simulink model "AUV_2DoF"  (R2020b)
settings: Solver=VariableStepAuto  StartTime=0.0  StopTime=60  RelTol=1e-3
libraries: pid_lib x4
settings Model: Creator=shanerutherford  LastModifiedBy=shanerutherford

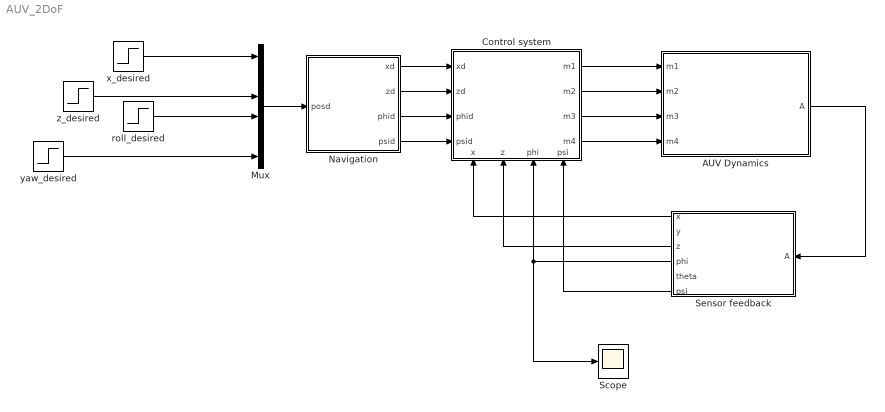
== system AUV_2DoF ==
  AUV Dynamics : Subsystem
  Control system : Subsystem
      settings: PortSchema="{\"entries\":[{\"content\":{\"sides\":[{\"content\":{\"connectorIds\":[\"In1\",\"In2\",\"In3\",\"In4\"]},\"type\":\"ConnectorPlacement.EquallySpacedRectSide\",\"uuid\":\"3eb5b42b-7b52-486e-935e-7444b7a9c48d\"},{\"content\":{\"connectorIds\":[\"Out1\",\"Out2\",\"Out3\",\"Out4\"],\"side\":\"RIGHT\"},\"type\":\"ConnectorPlacement.EquallySpacedRectSide\",\"uuid\":\"c474b75f-63e2-42a7-9927-f23487fa052b\"},{\"content\":{\"connectorIds\":[],\"side\":\"TOP\"},\"type\":\"ConnectorPlacement.EquallySpacedRectSide\",\"uuid\":\"fca6ae17-6a90-49a5-80ec-8d57e94c626d\"},{\"content\":{\"connectorIds\":[\"In5\",\"In6\",\"In7\",\"In8\"],\"side\":\"BOTTOM\"},\"type\":\"ConnectorPlacement.EquallySpacedRectSide\",\"uuid\":\"7c03cb94-1735-4782-aac2-3eb76e3c70ce\"},{\"content\":{\"connectorIds\":[],\"side\":\"HIDDEN\"},\"type\":\"ConnectorPlacement.EquallySpacedRectSide\",\"uuid\":\"5c2518b4-2d1f-408e-bcce-4e49db9481e4\"}]},\"type\":\"ConnectorPlacement.EquallySpacedConnector\",\"uuid\":\"da1a9c0d-6174-41ed-b6b8-df7c5a071ef3\"}],\"packageUris\":[\"http://schema.mathworks.com/mf0/Connector/R2020b\"],\"version\":\"1.0\"}"
  Mux : Mux  Inputs=6
  Navigation : MATLAB Function  TreatAsAtomicUnit=on
  Scope : Scope
  Sensor feedback : Subsystem
  roll_desired : Step  SampleTime=0
  x_desired : Step  After=0  SampleTime=0
  yaw_desired : Step  After=0  SampleTime=0
  z_desired : Step  After=0  SampleTime=0
  wires:
  Control system/1(m1) -> AUV Dynamics/1(m1)
  Control system/2(m2) -> AUV Dynamics/2(m2)
  Control system/3(m3) -> AUV Dynamics/3(m3)
  Control system/4(m4) -> AUV Dynamics/4(m4)
  AUV Dynamics/1(A) -> Sensor feedback/1(A)
  Sensor feedback/4(phi) -> Scope/1, Control system/7(phi)
  Sensor feedback/1(x) -> Control system/5(x)
  Sensor feedback/3(z) -> Control system/6(z)
  Sensor feedback/6(psi) -> Control system/8(psi)
  Navigation/1(xd) -> Control system/1(xd)
  Navigation/2(zd) -> Control system/2(zd)
  Navigation/3(phid) -> Control system/3(phid)
  Navigation/4(psid) -> Control system/4(psid)
  Mux/1 -> Navigation/1(posd)
  x_desired/1 -> Mux/1
  z_desired/1 -> Mux/3
  roll_desired/1 -> Mux/4
  yaw_desired/1 -> Mux/6

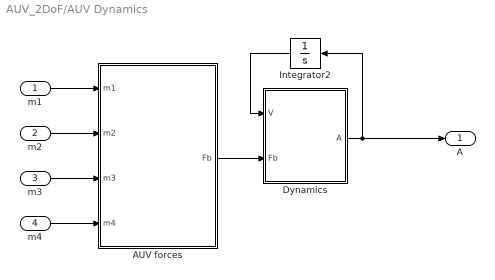
== system AUV_2DoF/AUV Dynamics ==
  m1 : Inport
  m2 : Inport  Port=2
  m3 : Inport  Port=3
  m4 : Inport  Port=4
  AUV forces : MATLAB Function  TreatAsAtomicUnit=on
  Dynamics : MATLAB Function  TreatAsAtomicUnit=on
  Integrator2 : Integrator
  A : Outport  PortDimensions=6
  wires:
  Dynamics/1(A) -> Integrator2/1, A/1
  m1/1 -> AUV forces/1(m1)
  m2/1 -> AUV forces/2(m2)
  m3/1 -> AUV forces/3(m3)
  m4/1 -> AUV forces/4(m4)
  AUV forces/1(Fb) -> Dynamics/2(Fb)
  Integrator2/1 -> Dynamics/1(V)

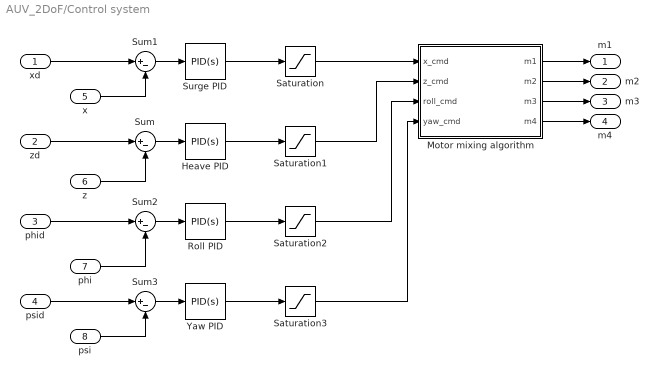
== system AUV_2DoF/Control system ==
  xd : Inport
  zd : Inport  Port=2
  phid : Inport  Port=3
  psid : Inport  Port=4
  x : Inport  Port=5
  z : Inport  Port=6
  phi : Inport  Port=7
  psi : Inport  Port=8
  Heave PID : pid_lib/PID Controller  Controller=PID  Form=Parallel  TimeDomain=Continuous-time  UseExternalTs=off  SampleTime=-1  IntegratorMethod=Forward Euler  FilterMethod=Forward Euler  ControllerParametersSource=internal  P=1  I=0  D=5  UseFilter=on  N=100  TunerSelectOption=Transfer Function Based (PID Tuner App)  InitialConditionSource=internal  InitialConditionForIntegrator=0  InitialConditionForFilter=0  DifferentiatorICPrevScaledInput=0  ExternalReset=none  TrackingMode=off  Kt=1  LimitOutput=off  SatLimitsSource=internal  UpperSaturationLimit=inf  LowerSaturationLimit=-inf  LinearizeAsGain=on  AntiWindupMode=none  Kb=1  POutMin=[]  POutMax=[]  IOutMin=[]  IOutMax=[]  DOutMin=[]  DOutMax=[]  NOutMin=[]  NOutMax=[]  SumOutMin=[]  SumOutMax=[]  SaturationOutMin=[]  SaturationOutMax=[]  PParamMin=[]  PParamMax=[]  IParamMin=[]  IParamMax=[]  DParamMin=[]  DParamMax=[]  NParamMin=[]  NParamMax=[]  KbParamMin=[]  KbParamMax=[]  KtParamMin=[]  KtParamMax=[]  KbOutMin=[]  KbOutMax=[]  KtOutMin=[]  KtOutMax=[]  IntegratorOutMin=[]  IntegratorOutMax=[]  FilterOutMin=[]  FilterOutMax=[]  SumI1OutMin=[]  SumI1OutMax=[]  SumI2OutMin=[]  SumI2OutMax=[]  SumI3OutMin=[]  SumI3OutMax=[]  SumI4OutMin=[]  SumI4OutMax=[]  SumDOutMin=[]  SumDOutMax=[]  DifferentiatorOutMin=[]  DifferentiatorOutMax=[]  FilterDiffOutCoefMin=[]  FilterDiffOutCoefMax=[]  ReciprocalOutMin=[]  ReciprocalOutMax=[]  SumDenOutMin=[]  SumDenOutMax=[]  SumNumOutMin=[]  SumNumOutMax=[]  DivideOutMin=[]  DivideOutMax=[]  UdiffTsProdOutMin=[]  UdiffTsProdOutMax=[]  NTsProdOutMin=[]  NTsProdOutMax=[]  UintegralTsProdOutMin=[]  UintegralTsProdOutMax=[]  UngainTsProdOutMin=[]  UngainTsProdOutMax=[]  IntegratorContinuousStateAttributes=''  IntegratorStateMustResolveToSignalObject=off  IntegratorRTWStateStorageClass=Auto  FilterContinuousStateAttributes=''  FilterStateMustResolveToSignalObject=off  FilterRTWStateStorageClass=Auto  ParallelPVariant=InternalParameters  IdealPVariant=Disabled  IVariant=InternalParameters  DVariant=InternalParameters  IntegratorVariant=Continuous  SatVariant=Disabled  AWVariant=Passthrough  PCopyVariant=Disabled  TRVariant=Disabled  FdbkBlocksVariant=Forward  IdealPFdbkVariant=Disabled  SatFdbkVariant=Disabled  DerivativeFilterVariant=ContFilter  NVariant=InternalParameters  NCopyVariant=Disabled  FilterICVariant=InternalICsFilter  IntegratorICVariant=InternalICs  ExternalResetVariant=Disabled  TRSumVariant=Passthrough  SumFdbkVariant=Disabled  SumVariant=Sum_PID  TsampFilterVariant=InternalTs  TsampNgainVariant=Passthrough  TsampIntegralVariant=Passthrough  ExternalSaturationOutDataTypeStr=Inherit: Same as second input
  Motor mixing algorithm : MATLAB Function  TreatAsAtomicUnit=on
  Roll PID : pid_lib/PID Controller  Controller=PID  Form=Parallel  TimeDomain=Continuous-time  UseExternalTs=off  SampleTime=-1  IntegratorMethod=Forward Euler  FilterMethod=Forward Euler  ControllerParametersSource=internal  P=1  I=0  D=5  UseFilter=on  N=100  TunerSelectOption=Transfer Function Based (PID Tuner App)  InitialConditionSource=internal  InitialConditionForIntegrator=0  InitialConditionForFilter=0  DifferentiatorICPrevScaledInput=0  ExternalReset=none  TrackingMode=off  Kt=1  LimitOutput=off  SatLimitsSource=internal  UpperSaturationLimit=inf  LowerSaturationLimit=-inf  LinearizeAsGain=on  AntiWindupMode=none  Kb=1  POutMin=[]  POutMax=[]  IOutMin=[]  IOutMax=[]  DOutMin=[]  DOutMax=[]  NOutMin=[]  NOutMax=[]  SumOutMin=[]  SumOutMax=[]  SaturationOutMin=[]  SaturationOutMax=[]  PParamMin=[]  PParamMax=[]  IParamMin=[]  IParamMax=[]  DParamMin=[]  DParamMax=[]  NParamMin=[]  NParamMax=[]  KbParamMin=[]  KbParamMax=[]  KtParamMin=[]  KtParamMax=[]  KbOutMin=[]  KbOutMax=[]  KtOutMin=[]  KtOutMax=[]  IntegratorOutMin=[]  IntegratorOutMax=[]  FilterOutMin=[]  FilterOutMax=[]  SumI1OutMin=[]  SumI1OutMax=[]  SumI2OutMin=[]  SumI2OutMax=[]  SumI3OutMin=[]  SumI3OutMax=[]  SumI4OutMin=[]  SumI4OutMax=[]  SumDOutMin=[]  SumDOutMax=[]  DifferentiatorOutMin=[]  DifferentiatorOutMax=[]  FilterDiffOutCoefMin=[]  FilterDiffOutCoefMax=[]  ReciprocalOutMin=[]  ReciprocalOutMax=[]  SumDenOutMin=[]  SumDenOutMax=[]  SumNumOutMin=[]  SumNumOutMax=[]  DivideOutMin=[]  DivideOutMax=[]  UdiffTsProdOutMin=[]  UdiffTsProdOutMax=[]  NTsProdOutMin=[]  NTsProdOutMax=[]  UintegralTsProdOutMin=[]  UintegralTsProdOutMax=[]  UngainTsProdOutMin=[]  UngainTsProdOutMax=[]  IntegratorContinuousStateAttributes=''  IntegratorStateMustResolveToSignalObject=off  IntegratorRTWStateStorageClass=Auto  FilterContinuousStateAttributes=''  FilterStateMustResolveToSignalObject=off  FilterRTWStateStorageClass=Auto  ParallelPVariant=InternalParameters  IdealPVariant=Disabled  IVariant=InternalParameters  DVariant=InternalParameters  IntegratorVariant=Continuous  SatVariant=Disabled  AWVariant=Passthrough  PCopyVariant=Disabled  TRVariant=Disabled  FdbkBlocksVariant=Forward  IdealPFdbkVariant=Disabled  SatFdbkVariant=Disabled  DerivativeFilterVariant=ContFilter  NVariant=InternalParameters  NCopyVariant=Disabled  FilterICVariant=InternalICsFilter  IntegratorICVariant=InternalICs  ExternalResetVariant=Disabled  TRSumVariant=Passthrough  SumFdbkVariant=Disabled  SumVariant=Sum_PID  TsampFilterVariant=InternalTs  TsampNgainVariant=Passthrough  TsampIntegralVariant=Passthrough  ExternalSaturationOutDataTypeStr=Inherit: Same as second input
  Saturation{,1..3} (4 alike) : Saturate  UpperLimit=0.3  LowerLimit=-0.3
  Sum{,1..3} (4 alike) : Sum  Inputs=|+-
  Surge PID : pid_lib/PID Controller  Controller=PID  Form=Parallel  TimeDomain=Continuous-time  UseExternalTs=off  SampleTime=-1  IntegratorMethod=Forward Euler  FilterMethod=Forward Euler  ControllerParametersSource=internal  P=1  I=0  D=5  UseFilter=on  N=100  TunerSelectOption=Transfer Function Based (PID Tuner App)  InitialConditionSource=internal  InitialConditionForIntegrator=0  InitialConditionForFilter=0  DifferentiatorICPrevScaledInput=0  ExternalReset=none  TrackingMode=off  Kt=1  LimitOutput=off  SatLimitsSource=internal  UpperSaturationLimit=inf  LowerSaturationLimit=-inf  LinearizeAsGain=on  AntiWindupMode=none  Kb=1  POutMin=[]  POutMax=[]  IOutMin=[]  IOutMax=[]  DOutMin=[]  DOutMax=[]  NOutMin=[]  NOutMax=[]  SumOutMin=[]  SumOutMax=[]  SaturationOutMin=[]  SaturationOutMax=[]  PParamMin=[]  PParamMax=[]  IParamMin=[]  IParamMax=[]  DParamMin=[]  DParamMax=[]  NParamMin=[]  NParamMax=[]  KbParamMin=[]  KbParamMax=[]  KtParamMin=[]  KtParamMax=[]  KbOutMin=[]  KbOutMax=[]  KtOutMin=[]  KtOutMax=[]  IntegratorOutMin=[]  IntegratorOutMax=[]  FilterOutMin=[]  FilterOutMax=[]  SumI1OutMin=[]  SumI1OutMax=[]  SumI2OutMin=[]  SumI2OutMax=[]  SumI3OutMin=[]  SumI3OutMax=[]  SumI4OutMin=[]  SumI4OutMax=[]  SumDOutMin=[]  SumDOutMax=[]  DifferentiatorOutMin=[]  DifferentiatorOutMax=[]  FilterDiffOutCoefMin=[]  FilterDiffOutCoefMax=[]  ReciprocalOutMin=[]  ReciprocalOutMax=[]  SumDenOutMin=[]  SumDenOutMax=[]  SumNumOutMin=[]  SumNumOutMax=[]  DivideOutMin=[]  DivideOutMax=[]  UdiffTsProdOutMin=[]  UdiffTsProdOutMax=[]  NTsProdOutMin=[]  NTsProdOutMax=[]  UintegralTsProdOutMin=[]  UintegralTsProdOutMax=[]  UngainTsProdOutMin=[]  UngainTsProdOutMax=[]  IntegratorContinuousStateAttributes=''  IntegratorStateMustResolveToSignalObject=off  IntegratorRTWStateStorageClass=Auto  FilterContinuousStateAttributes=''  FilterStateMustResolveToSignalObject=off  FilterRTWStateStorageClass=Auto  ParallelPVariant=InternalParameters  IdealPVariant=Disabled  IVariant=InternalParameters  DVariant=InternalParameters  IntegratorVariant=Continuous  SatVariant=Disabled  AWVariant=Passthrough  PCopyVariant=Disabled  TRVariant=Disabled  FdbkBlocksVariant=Forward  IdealPFdbkVariant=Disabled  SatFdbkVariant=Disabled  DerivativeFilterVariant=ContFilter  NVariant=InternalParameters  NCopyVariant=Disabled  FilterICVariant=InternalICsFilter  IntegratorICVariant=InternalICs  ExternalResetVariant=Disabled  TRSumVariant=Passthrough  SumFdbkVariant=Disabled  SumVariant=Sum_PID  TsampFilterVariant=InternalTs  TsampNgainVariant=Passthrough  TsampIntegralVariant=Passthrough  ExternalSaturationOutDataTypeStr=Inherit: Same as second input
  Yaw PID : pid_lib/PID Controller  Controller=PID  Form=Parallel  TimeDomain=Continuous-time  UseExternalTs=off  SampleTime=-1  IntegratorMethod=Forward Euler  FilterMethod=Forward Euler  ControllerParametersSource=internal  P=1  I=0  D=5  UseFilter=on  N=100  TunerSelectOption=Transfer Function Based (PID Tuner App)  InitialConditionSource=internal  InitialConditionForIntegrator=0  InitialConditionForFilter=0  DifferentiatorICPrevScaledInput=0  ExternalReset=none  TrackingMode=off  Kt=1  LimitOutput=off  SatLimitsSource=internal  UpperSaturationLimit=inf  LowerSaturationLimit=-inf  LinearizeAsGain=on  AntiWindupMode=none  Kb=1  POutMin=[]  POutMax=[]  IOutMin=[]  IOutMax=[]  DOutMin=[]  DOutMax=[]  NOutMin=[]  NOutMax=[]  SumOutMin=[]  SumOutMax=[]  SaturationOutMin=[]  SaturationOutMax=[]  PParamMin=[]  PParamMax=[]  IParamMin=[]  IParamMax=[]  DParamMin=[]  DParamMax=[]  NParamMin=[]  NParamMax=[]  KbParamMin=[]  KbParamMax=[]  KtParamMin=[]  KtParamMax=[]  KbOutMin=[]  KbOutMax=[]  KtOutMin=[]  KtOutMax=[]  IntegratorOutMin=[]  IntegratorOutMax=[]  FilterOutMin=[]  FilterOutMax=[]  SumI1OutMin=[]  SumI1OutMax=[]  SumI2OutMin=[]  SumI2OutMax=[]  SumI3OutMin=[]  SumI3OutMax=[]  SumI4OutMin=[]  SumI4OutMax=[]  SumDOutMin=[]  SumDOutMax=[]  DifferentiatorOutMin=[]  DifferentiatorOutMax=[]  FilterDiffOutCoefMin=[]  FilterDiffOutCoefMax=[]  ReciprocalOutMin=[]  ReciprocalOutMax=[]  SumDenOutMin=[]  SumDenOutMax=[]  SumNumOutMin=[]  SumNumOutMax=[]  DivideOutMin=[]  DivideOutMax=[]  UdiffTsProdOutMin=[]  UdiffTsProdOutMax=[]  NTsProdOutMin=[]  NTsProdOutMax=[]  UintegralTsProdOutMin=[]  UintegralTsProdOutMax=[]  UngainTsProdOutMin=[]  UngainTsProdOutMax=[]  IntegratorContinuousStateAttributes=''  IntegratorStateMustResolveToSignalObject=off  IntegratorRTWStateStorageClass=Auto  FilterContinuousStateAttributes=''  FilterStateMustResolveToSignalObject=off  FilterRTWStateStorageClass=Auto  ParallelPVariant=InternalParameters  IdealPVariant=Disabled  IVariant=InternalParameters  DVariant=InternalParameters  IntegratorVariant=Continuous  SatVariant=Disabled  AWVariant=Passthrough  PCopyVariant=Disabled  TRVariant=Disabled  FdbkBlocksVariant=Forward  IdealPFdbkVariant=Disabled  SatFdbkVariant=Disabled  DerivativeFilterVariant=ContFilter  NVariant=InternalParameters  NCopyVariant=Disabled  FilterICVariant=InternalICsFilter  IntegratorICVariant=InternalICs  ExternalResetVariant=Disabled  TRSumVariant=Passthrough  SumFdbkVariant=Disabled  SumVariant=Sum_PID  TsampFilterVariant=InternalTs  TsampNgainVariant=Passthrough  TsampIntegralVariant=Passthrough  ExternalSaturationOutDataTypeStr=Inherit: Same as second input
  m1 : Outport
  m2 : Outport  Port=2
  m3 : Outport  Port=3
  m4 : Outport  Port=4
  wires:
  psid/1 -> Sum3/1
  Yaw PID/1 -> Saturation3/1
  Sum2/1 -> Roll PID/1
  Saturation/1 -> Motor mixing algorithm/1(x_cmd)
  zd/1 -> Sum/1
  x/1 -> Sum1/2
  Sum1/1 -> Surge PID/1
  Sum/1 -> Heave PID/1
  Roll PID/1 -> Saturation2/1
  xd/1 -> Sum1/1
  psi/1 -> Sum3/2
  Saturation2/1 -> Motor mixing algorithm/3(roll_cmd)
  phid/1 -> Sum2/1
  Sum3/1 -> Yaw PID/1
  Saturation3/1 -> Motor mixing algorithm/4(yaw_cmd)
  Saturation1/1 -> Motor mixing algorithm/2(z_cmd)
  z/1 -> Sum/2
  Surge PID/1 -> Saturation/1
  Heave PID/1 -> Saturation1/1
  phi/1 -> Sum2/2
  Motor mixing algorithm/1(m1) -> m1/1
  Motor mixing algorithm/2(m2) -> m2/1
  Motor mixing algorithm/3(m3) -> m3/1
  Motor mixing algorithm/4(m4) -> m4/1

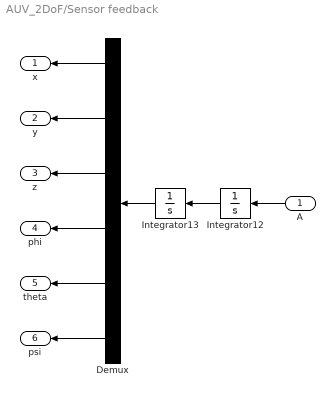
== system AUV_2DoF/Sensor feedback ==
  A : Inport
  Demux : Demux  Outputs=6
  Integrator12 : Integrator
  Integrator13 : Integrator
  x : Outport
  y : Outport  Port=2
  z : Outport  Port=3
  phi : Outport  Port=4
  theta : Outport  Port=5
  psi : Outport  Port=6
  wires:
  Demux/2 -> y/1
  Demux/1 -> x/1
  Demux/3 -> z/1
  Demux/4 -> phi/1
  Demux/5 -> theta/1
  Demux/6 -> psi/1
  Integrator12/1 -> Integrator13/1
  Integrator13/1 -> Demux/1
  A/1 -> Integrator12/1

== matlab function AUV_2DoF/Control system/Motor mixing algorithm ==
  data: x_cmd input; m1 output; z_cmd input; m2 output; m3 output; m4 output; roll_cmd input; yaw_cmd input
function [m1, m2, m3, m4] = fcn(x_cmd, z_cmd, roll_cmd, yaw_cmd)

% m1 m2 m3 and m4 are front-right, front-left, back-right and back-left
% motors respectively

    function [min] = abs_min(v1, v2)
        if abs(v1) < abs(v2) 
            min = v1;
        else
            min = v2;
        end
    end

max_response = 50;

m1 = abs_min(-z_cmd - roll_cmd, max_response);
m2 = abs_min(-z_cmd + roll_cmd, max_response);
m3 = abs_min(x_cmd - yaw_cmd, max_response);
m4 = abs_min(x_cmd + yaw_cmd, max_response);
end

== matlab function AUV_2DoF/Navigation ==
  data: posd input; xd output; zd output; phid output; psid output
function [xd, zd, phid, psid] = fcn(posd)

xd = posd(1);
zd = posd(3);
phid = posd(4);
psid = posd(6);

== matlab function AUV_2DoF/AUV Dynamics/AUV forces ==
  data: Fb output; m1 input; m2 input; m3 input; m4 input
function Fb = fcn(m1, m2, m3, m4)

% x, y and z axis relates to local front (bow), starboard and down
% directions
% phi, theta and psi represents roll, pitch and yaw respectivly

% assuming that the force produced by each motor is proportonal to the
% signal voltage
thrust_constant = 1;
roll_constant = 1;
yaw_constant = 1;

Fb = [
    thrust_constant*(m3+m4) 
    0                           % AUV cannot move in y direction
    -thrust_constant*(m1+m2)    % positive z is downward 
    roll_constant*(m2-m1)       % positive rotation is clockwise
    0                           % AUV cannot pitch 
    yaw_constant*(m4-m3)
];

== matlab function AUV_2DoF/AUV Dynamics/Dynamics ==
  data: V input; Fb input; A output
function A = fcn(V, Fb)

mass = 10;
F_resistance = V.^2;
A = (Fb - F_resistance)./mass;
